simulink model "acc"  (R2021b)
settings: Solver=FixedStepAuto  StartTime=0.0  StopTime=206  FixedStep=0.0005  RelTol=1e-3
values from neighbouring files (symbols this model uses):
  Leftdis_PV_switch = 2    [acc_plot_backup.m]
  s_path = [0 1.10508939428 2.2141958029 3.32141571172 4.42705301151 5.53154548532 6.63517443471 7.73808041313 8.84055018688 9.94289959674 11.0453539299 12.1480581097 ... (1001 elements, 1001x1)]    [200_100radius.mat]    (also in LV_Clothoid_S_Turn_path.mat = [0 0.966832089581 1.93621320584 2.90214024471 3.86476766313 ; NEDC_path.mat = [0 0.414605943146 0.832514087334 1.25401518562 1.68216660344; Straight_East_into_curve.mat = [0 1.65770560069 3.32192925577 4.98420060507 6.64484613518 8; acc_plot_backup.m = Station_HV_m)
  X_path = [0 1.10508939428 2.2141958029 3.32141571172 4.42705301151 5.53154548532 6.63517443471 7.73808041313 8.84055018688 9.94289959674 11.0453539299 12.1480581097 ... (1001 elements, 1001x1)]    [200_100radius.mat]    (also in LV_Clothoid_S_Turn_path.mat = [-10 -9.03316791042 -8.06378679416 -7.09785975529 -6.1352323; NEDC_path.mat = [0 0.414605943146 0.832514087334 1.25401518562 1.68216660344; Straight_East_into_curve.mat = [0 1.65770560069 3.32192925577 4.98420060507 6.64484613518 8; acc_plot_backup.m = X_HV_m)
  Y_path = [0 -1.70364610795e-18 -7.41532896709e-18 1.46822109542e-17 4.74557362791e-17 6.12980216762e-17 9.25043977736e-17 1.24088240159e-16 1.5099156923e-16 1.7058517853e-16 1.90629227614e-16 2.09673434424e-16 ... (1001 elements, 1001x1)]    [200_100radius.mat]    (also in LV_Clothoid_S_Turn_path.mat = [0 -8.46153035536e-19 5.07382551045e-18 2.07356032218e-17 3.; NEDC_path.mat = [0 -3.50680326162e-18 -2.14111304971e-18 3.38197671014e-18 3; Straight_East_into_curve.mat = [0 1.29197709199e-18 2.81882429322e-18 3.49020462564e-17 6.7; acc_plot_backup.m = Y_HV_m)
undefined symbols (not defined in the file or in its folder): C_TICK_TIME_S, ENUM_ACCSTATE_DISABLED, ENUM_ACCSTATE_OFF, ENUM_ACCSTATE_STANDBY, FALSE, KVDI_ACCLongPressTime_ms, KVDI_ACCMaxActSpeed_kph, KVDI_ACCSetSpdIntial_kph, KVDI_ACCSpdLargeChange_kph, KVDI_LongPressConTime_ms, ONE_FLOAT, ONE_INT, R, Rw, T, TRUE, ZERO_FLOAT, ZERO_INT
libraries: simulink x16, dspstat3 x4, simulink_extras x2, Solver_SF x1
(part 4 of 4)

== matlab function acc/relative_dynamic_estimated/Measurement_update_X2 ==
  data: X_e input; u input; X_b output
function X_b=fcn(X_e,u)
T=0.01;
F=[1 T 0.5*T^2;0 1 T;0 0 1];
G=[-1/6*T^3;-1/2*T^2;-T];

X_b=F*X_e+G*u;
end

== matlab function acc/relative_dynamic_estimated/Time_update_X2 ==
  data: R input; Q input; K output; M2 output; M input
function [K,M2] = fcn(R,Q,M)
T=0.01;
% Rw=0.8;
% R=0.0001;
F=[1 T 0.5*T^2;0 1 T;0 0 1];
H=[1 0 0];
G=[-1/6*T^3;-1/2*T^2;-T];
G2=[1/6*T^3;1/2*T^2;T];

P=M-M*H'*inv(H*M*H'+R)*H*M;
% M2=F*P*F'+G2*Rw*G2';
M2=F*P*F'+Q;
K=P*H'*inv(R);
end

== matlab function acc/relative_dynamic_estimated/MATLAB Function3 ==
  data: X_b input; X_e output; K input; y input; d output; e output
function [X_e,d,e] = fcn(X_b,K,y)
H=[1 0 0];
d=y-H*X_b;
X_e=X_b+K*(y-H*X_b);
e=y-H*X_e;
end

== matlab function acc/relative_dynamic_estimated/MATLAB Function4 ==
  data: Q input; Q2 output; R input; M input; e input; d input; K input; R2 output; G output
function [Q2,R2,G] = fcn(Q,R,M,e,d,K)
a=0.9;
b=0.9;
H=[1 0 0];
R2=a*R+(1-a)*(e*e'+H*M*H');

Q2=b*Q+2*(1-b)*(K*d*d'*K');
G=0*Q+K*d*d*K';
end

== matlab function acc/relative_dynamic_estimated/Measurement_update_X3 ==
  data: X_e input; u input; X_b output
function X_b=fcn(X_e,u)
T=0.01;
F=[1 T 0.5*T^2;0 1 T;0 0 1];
G=[-1/6*T^3;-1/2*T^2;-T];

X_b=F*X_e+G*u;
end

== matlab function acc/relative_dynamic_estimated/Time_update_X3 ==
  data: R input; Q input; K output; M2 output; M input
function [K,M2] = fcn(R,Q,M)
T=0.01;
% Rw=0.8;
% R=0.0001;
F=[1 T 0.5*T^2;0 1 T;0 0 1];
H=[1 0 0];
G=[-1/6*T^3;-1/2*T^2;-T];
G2=[1/6*T^3;1/2*T^2;T];

P=M-M*H'*inv(H*M*H'+R)*H*M;
% M2=F*P*F'+G2*Rw*G2';
M2=F*P*F'+Q;
K=P*H'*inv(R);
end

== matlab function acc/Subsystem/longitudinal_driver_reference7 ==
  data: longitudinal_lane_refernce_trigger input; T input; Vxo input; Vxt input; ax_max input; jx_max input; Vx output; t output
function [Vx,t] = fcn(longitudinal_lane_refernce_trigger,T,Vxo,Vxt,ax_max,jx_max)
Vx=0;
Ax=0;
t=0;

if Vxt < Vxo
    ax_max=-ax_max;
    jx_max=-jx_max;
end

if longitudinal_lane_refernce_trigger==1

t1=ax_max/jx_max;
t2=(Vxt-Vxo)/ax_max;
t3=t1+t2;
t=T+0.1;


V1=Vxo+(0.5*jx_max*(t1^2));
V2=V1+(ax_max*(t2-t1));
   if t>=0 && t<=t1
       Ax=jx_max*t;
       Vx=double(Vxo+0.5*jx_max*(t^2));
   end
   if t>t1 && t<=t2
       Ax=ax_max;
       Vx=double(V1+(ax_max*(t-t1)));
   end
   if t>t2 && t<=t3
       Ax=ax_max-(jx_max*(t-t2));
       Vx=double(V2+ax_max*(t-t2)-0.5*jx_max*((t-t2)^2));
   end
   if t>t3
       Vx=double(Vxt);
       Ax=0;
   end
       

end
if longitudinal_lane_refernce_trigger==0
  Vx=double(Vxo);
 

   
end
end

== matlab function acc/Subsystem/longitudinal_driver_reference8 ==
  data: longitudinal_lane_refernce_trigger input; T input; Vxo input; Vxt input; ax_max input; jx_max input; Vx output; t output
function [Vx,t] = fcn(longitudinal_lane_refernce_trigger,T,Vxo,Vxt,ax_max,jx_max)
Vx=0;
Ax=0;
t=0;

if Vxt < Vxo
    ax_max=-ax_max;
    jx_max=-jx_max;
end

if longitudinal_lane_refernce_trigger==1

t1=ax_max/jx_max;
t2=(Vxt-Vxo)/ax_max;
t3=t1+t2;
t=T+0.1;


V1=Vxo+(0.5*jx_max*(t1^2));
V2=V1+(ax_max*(t2-t1));
   if t>=0 && t<=t1
       Ax=jx_max*t;
       Vx=double(Vxo+0.5*jx_max*(t^2));
   end
   if t>t1 && t<=t2
       Ax=ax_max;
       Vx=double(V1+(ax_max*(t-t1)));
   end
   if t>t2 && t<=t3
       Ax=ax_max-(jx_max*(t-t2));
       Vx=double(V2+ax_max*(t-t2)-0.5*jx_max*((t-t2)^2));
   end
   if t>t3
       Vx=double(Vxt);
       Ax=0;
   end
       

end
if longitudinal_lane_refernce_trigger==0
  Vx=double(Vxo);
 

   
end
end

== matlab function acc/Camera_NEW ==
  data: ux_mps input; phi_deg input; Xo input; Yo input; X_path parameter; s_path parameter; station input; x_ref output size=[22 1]; y_ref output size=[22 1]; Heading_ref output size=[22 1]; C output; Y_path parameter; Ts_MPC input
function [x_ref,y_ref,Heading_ref,C]  = Camera_emulator(ux_mps,phi_deg,Xo,Yo, X_path, s_path,station,Y_path, Ts_MPC)
% function [x_ref,y_ref,Y_path,Heading_ref,C]  = Camera_emulator(ux_mps,phi_deg,Xo,Yo, X_path, s_path,station,t_start,Ts_MPC,AES_pre_time,speed,Np,C0_Old, Y_path_Old)
% Path information is X_path, Y_path, s_path 
% Load path before running model===========================================
Np=22;
Tp=Ts_MPC*Np;

phi_rad=phi_deg*pi/180;

% global reference
% Yr=interp1(s_path,Y_path,station);
% path x,y body coordinate=================================================
x_path=cos(phi_rad)*(X_path-Xo)+sin(phi_rad)*(Y_path-Yo);
y_path=-sin(phi_rad)*(X_path-Xo)+cos(phi_rad)*(Y_path-Yo);
% current x,y body coordinate
% x_ref(1)=interp1(s_path,x_path,station);
% y_ref(1)=interp1(s_path,y_path,station);

s=ones(Np+2,1);
delta_s=Ts_MPC*ux_mps;
s=diag(0:Np+1)*s*delta_s+station;
%s=diag(-1:Np)*s*delta_s+station;

x_ref=zeros(Np,1);
y_ref=zeros(Np,1);
x_ref_12=interp1(s_path,x_path,s);
y_ref_12=interp1(s_path,y_path,s);
x_ref=x_ref_12(2:Np+1);
y_ref=y_ref_12(2:Np+1);
s_temp=s(Np)+Ts_MPC*ux_mps;

Heading_ref=zeros(Np,1);
for i=1:Np
    Heading_ref(i)=atan2(y_ref_12(i+2)-y_ref_12(i+1),x_ref_12(i+2)-x_ref_12(i+1));
end


%% CR=polyfit(x_R,y_R,3);
x=x_ref;
% Lane Change Module ======================================================

% if y_ref >= 1.5
%     y=y_ref-3.66;
% elseif y_ref <= -1.5
%     y=y_ref+3.66;
% else
%     y=y_ref+0;
% end
if y_ref >= 1.5
    y=y_ref-3.66;
elseif y_ref <= -1.5
    y=y_ref+3.66;
else
    y=y_ref+0;
end

%===================================================================
sum_x1=sum(x);
sum_x2=sum(x.^2);
sum_x3=sum(x.^3);
sum_x4=sum(x.^4);
sum_x5=sum(x.^5);
sum_x6=sum(x.^6);
sum_y=sum(y);
A=[length(x) sum_x1 sum_x2 sum_x3;
        sum_x1 sum_x2 sum_x3 sum_x4; 
        sum_x2 sum_x3 sum_x4 sum_x5; 
        sum_x3 sum_x4 sum_x5 sum_x6];
% A=[50 sum_x1 sum_x2 sum_x3;
%         sum_x1 sum_x2 sum_x3 sum_x4; 
%         sum_x2 sum_x3 sum_x4 sum_x5; 
%         sum_x3 sum_x4 sum_x5 sum_x6];
B=[sum_y;
      sum(x.*y);
      sum(x.*x.*y);
      sum(x.*x.*x.*y)];
% AES_pre_time=5;
% if Xo<=speed/3.6*(t_start-AES_pre_time)
%     C=[0; 0; 0; 0];
% else
    C=inv(A)*B;
% end
end

== matlab function acc/MPC_ACC ==
  data: trig input; vx_p input; u output; Vx input; ax input; Qs input; Rs input
function u = fcn(trig,vx_p,Vx,ax,Qs,Rs)
%% Initialzization
T = 0.1;
tau = 0.3;
Np = 10;
Nc = 3;

%% Mode Selector && MPC

A_spd = [1 T;0 1-T/tau];
B_spd = [0;T/tau];
C_spd = [1 0];

if trig == 1
    [m1,n1] = size(C_spd);
    h = zeros(Np,n1);
    F = zeros(Np,n1);
    h(1,:)=C_spd;
    F(1,:)=C_spd*A_spd;
    for j=2:Np
    h(j,:)=h(j-1,:)*A_spd; %Phi
    F(j,:)= F(j-1,:)*A_spd; 
    end
    v = h*B_spd;
    Phi_vx = zeros(Np,Nc);
    Phi_vx(:,1) = v;
    for k = 2:Nc
       Phi_vx(:,k) = [zeros(k-1,1);v(1:Np-k+1,1)]; %Toeplitz matrix
    end
    Q=Qs.*eye(Np); %Qw權重值=1;10
    R=Rs.*eye(Nc);%Rw權重值=0.07;1.5 ,0.07
    
    x_spd = [Vx;ax];
    Yref = vx_p';
    
    H = Phi_vx'*Q*Phi_vx+R;
    f = Phi_vx'*Q*(Yref-F*x_spd);
    U = inv(H)*f;
    u = U(1);

else
    u=0;
end
end

== matlab function acc/MATLAB Function5 ==
  data: u input; y output
function y = fcn(u)
persistent i;
if isempty(i)
    i = 1;
end

if i >=length(u)
    i=length(u);
end

y = u(i);
i = i+1;

== matlab function acc/MATLAB Function13 ==
  data: u input; y output
function y = fcn(u)
persistent i;
if isempty(i)
    i = 1;
end

if i >=length(u)
    i=length(u);
end

y = u(i);
i = i+1;

== matlab function acc/relative_dynamic_estimated/MATLAB Function6 ==
  data: X_b input; X_e output; K input; y input; d output; e output
function [X_e,d,e] = fcn(X_b,K,y)
H=[1 0 0];
d=y-H*X_b;
X_e=X_b+K*d;
e=y-H*X_e;
end

== matlab function acc/relative_dynamic_estimated/MATLAB Function7 ==
  data: Q input; Q2 output; R input; M input; e input; d input; K input; R2 output
function [Q2,R2] = fcn(Q,R,M,e,d,K)
a=0.5;
b=1;
H=[1 0 0];
R2=a*R+(1-a)*(e*e'+H*M*H');
if abs(d) < 0.02
    Q2=Q;
else
    Q2=b*Q+(1-b)*(K*d*d'*K');
end
end

== matlab function acc/relative_dynamic_estimated/Measurement_update_X5 ==
  data: X_e input; u input; X_b output
function X_b=fcn(X_e,u)
T=0.1;
F=[1 T 0.5*T^2;0 1 T;0 0 1];
G=[-1/6*T^3;-1/2*T^2;-T];

X_b=F*X_e+G*u;
end

== matlab function acc/relative_dynamic_estimated/Time_update_X5 ==
  data: R input; Q input; K output; M2 output; M input
function [K,M2] = fcn(R,Q,M)
T=0.1;
%% normal Kalman filter
% Rw=1; %變速度
% R=0.0001;
% Rw=0.5; %定速80
% R=0.001;
%% Adptive Kalman filter
%% 參數
F=[1 T 0.5*T^2;0 1 T;0 0 1];
H=[1 0 0];
G=[-(T^3)/6;-(T^2)/2;-T];
G2=[(T^3)/6;(T^2)/2;T];
%%
P=M-M*H'*inv(H*M*H'+R)*H*M;
% M2=F*P*F'+G2*Rw*G2';
M2=F*P*F'+Q;
K=P*H'*inv(R);
end

== matlab function acc/relative_dynamic_estimated/Q1 ==
  data: Rw output; d input; dx input; Rw1 input
function Rw  = fcn(d,dx,Rw1)
g=abs(d-dx);
if g > 0.04 && g< 0.5
    t=5;
elseif g <= 0.04 && g>0.02
    t=2;
else
    t=1;
end
if abs(d) > 0.002
    Rw=0.4*Rw1+0.6*abs(d^2)*10^t;
else
    Rw=Rw1*0.5;
end

end

== matlab function acc/relative_dynamic_estimated/R ==
  data: R output; e input; M input; R1 input
function R  = fcn(e,M,R1)
H=[1 0 0];
    R=(0.3*R1+0.7*(e*e+H*(M)*H'))/10;

end

== matlab function acc/relative_dynamic_estimated/Time_update_X6 ==
  data: Q input; R input; K output; P output; M2 output; M input
function [K,P,M2] = fcn(Q,R,M)
T=0.1;
% Rw=1; %變速度
% R=0.0001;
% Rw=1; %定速80
% R=0.001;
F=[1 T 0.5*T^2;0 1 T;0 0 1];
H=[1 0 0];
G=[-(T^3)/6;-(T^2)/2;-T];
G2=[(T^3)/6;(T^2)/2;T];

P=M-M*H'*inv(H*M*H'+R)*H*M;
M2=F*P*F'+G2*Q*G2';
% M2=F*P*F'+Q;
K=P*H'*inv(R);
end

== matlab function acc/relative_dynamic_estimated/Q ==
  data: Q output; d input; K input; Q1 input
function Q  = fcn(d,K,Q1)
if abs(d) > 0.002
    Q=0.3*Q1+0.7*(K*d*d*K');
else
    Q=Q1*0.9;
end

end

== matlab function acc/relative_dynamic_estimated/R2 ==
  data: R output; e input; M input; R1 input
function R  = fcn(e,M,R1)
H=[1 0 0];
% if e < 0.000001
%     R=R1;
% else
if abs(e)>0.1
    e=0.1;
end

% if abs(e) > 0.01
    R=0.3*R1+0.7*(e*e'+H*(M)*H');
%     R=0.3*R1+0.7*(e*e'+H*(M)*H')/;
% else
%     R=R1;
% end
% end
%     if R>0.01
%         R=0.01;
%     end
end

== matlab function acc/Subsystem/longitudinal_driver_reference9 ==
  data: longitudinal_lane_refernce_trigger input; T input; Vxo input; Vxt input; ax_max input; jx_max input; Vx output; t output
function [Vx,t] = fcn(longitudinal_lane_refernce_trigger,T,Vxo,Vxt,ax_max,jx_max)
Vx=0;
Ax=0;
t=0;

if Vxt < Vxo
    ax_max=-ax_max;
    jx_max=-jx_max;
end

if longitudinal_lane_refernce_trigger==1

t1=ax_max/jx_max;
t2=(Vxt-Vxo)/ax_max;
t3=t1+t2;
t=T+0.1;


V1=Vxo+(0.5*jx_max*(t1^2));
V2=V1+(ax_max*(t2-t1));
   if t>=0 && t<=t1
       Ax=jx_max*t;
       Vx=double(Vxo+0.5*jx_max*(t^2));
   end
   if t>t1 && t<=t2
       Ax=ax_max;
       Vx=double(V1+(ax_max*(t-t1)));
   end
   if t>t2 && t<=t3
       Ax=ax_max-(jx_max*(t-t2));
       Vx=double(V2+ax_max*(t-t2)-0.5*jx_max*((t-t2)^2));
   end
   if t>t3
       Vx=double(Vxt);
       Ax=0;
   end
       

end
if longitudinal_lane_refernce_trigger==0
  Vx=double(Vxo);
 

   
end
end

== matlab function acc/Estimation_TTCx_PV ==
  data: R input; TTC1 output; V input; A input; TTC2 output
function [TTC1,TTC2] = TTCx(R,V,A)
TTCp1=10;
TTCp2=10;
if R < 0
    R=-R;
    V=-V;
    A=-A;
end
% if R > 7
%     R=R-7;
% else
%     R=0;
% end
if R <= 0.1 % buff
    TTC1=0;
else
    if abs(A) > 1 && (V^2-2*A*R)>0
        TTCp1=(-V+sqrt(V^2-2*A*R))/A;
        TTCp2=(-V-sqrt(V^2-2*A*R))/A;
        if TTCp1>0 && TTCp2 >0
            TTC1 =min(TTCp1,TTCp2);
        elseif TTCp1 >= 0
            TTC1=TTCp1;
        else
            TTC1=TTCp2;
        end
    else
    TTC1=-R/V;
    end
end

if TTC1 > 10 
    TTC1=10;
end
if TTC1 < 0 
    TTC1=10;
end

if R < 0.1
    TTC2=0;
else
    TTC2=-R/V;
end
if  TTC2 > 10
    TTC2=10;
end
if  TTC2 < 0
    TTC2=10;
end
end

== matlab function acc/MPC_Bicycle_LDC1 ==
  data: trig input; Yref input; u output; Qs input; Rs input; Vy input; yaw_rate input; steer_angel input; Vx input; Ax input
function u  = fcn(trig,Yref,Qs,Rs,Vy,yaw_rate,steer_angel,Vx,Ax)
%% parameter
m=1501;
Caf=80.03*10^3;
Car=80.49*10^3;
Iz=1536.7; %2315
a=1.015;
b=1.895;
Np=10;
Nc=3;
tau=0.3;
T=0.1;
Y_ref=Yref;


if trig ==1


%% vehicle parameter

vx=zeros(Np,1);
vx(1)=Vx;
for z=2:Np
    vx(z)=vx(z-1)+Ax*T;
end

x_state = [0,Vy,0,yaw_rate,steer_angel]';



%% Vehicle Kinematics Model
% ----------------------------------------%
% x = [y, yaw angle, steering wheel angle]
% state row =5, state column =5,
%-----------------------------------------%
sr =5;
sc =5;
B = [0 0 0 0 (1/tau)*T]';
H = [1 0 0 0 0]; % [1, sr]

%% MPC parameter
% ------------------------------------------------------------------------------------------%
% Am is a vertor [A(k); A(k+1); A(k+2) ... A(k+np-1)]
% ------------------------------------------------------------------------------------------%
Am = zeros(sr, sc, Np);
for i = 1 : Np
    a13=vx(i)*T;
    a22=1-(Caf+Car)*T/(m*vx(i));
    a24=(b*Car-a*Caf)*T/(m*vx(i))-vx(i)*T;
    a25=Caf*T/m;
    a42=(b*Car-a*Caf)*T/(Iz*vx(i));
    a44=1-((a^2)*Caf+(b^2)*Car)*T/(Iz*vx(i));
    a45=a*Caf*T/Iz;
    a55=1-T/tau;
    Am(:,:,i)=[1 T a13 0 0;
        0 a22 0 a24 a25
        0 0 1 T 0
        0 a42 0 a44 a45
        0 0 0 0 a55];
end
% ------------------------------------------------------------------------------------------%
% Amm is a vector [A(k); A(k)A(k+1); A(k)A(k+1)A(k+2) ... A(k+np-1)]
% ------------------------------------------------------------------------------------------%
Amm = zeros(sr, sc, Np);
Amm(:, :, 1) = Am(:, :, 1);
for i = 2 : Np
    Amm(:, :, i) = Am(:, :, i) * Amm(:, :, i - 1);
end
% ----------------------------------------------------------------------------------------------%
% F is a metric [H A(k); H A(k)A(k+1); H A(k)A(k+1)A(k+2) ... H A(k+np-1)]
% size = [np, sc]
% ----------------------------------------------------------------------------------------------%
F = zeros(Np, sc);
for i = 1 : Np
    F(i, :) = H * Amm(:, : ,i);
end

% ----------------------------------------------------------------------------------------------%
% K is a metric [H A(k); H A(k)A(k+1); H A(k)A(k+1)A(k+2) ... H A(k+np-1)]
%size = [np nc]
%[H*B                                 0             0  ...       0  ]
%[H*A(k)*B                       H*B          0  ...        0 ] 
%[H*A(k)*A(k+1)*B       H*A(k)*B      0  ...    H*B ]
% the following quation is modified

%[H*B                                 0                   0          0          ...           0 ]
%[H*A(k+1)*B                          H*B                 0          0          ...           0 ] 
%[H*A(k+2)*A(k+1)*B                 H*A(k+2)*B           H*B         0          ...           0 ]
%[H*A(k+3)*A(k+2)*A(k+1)*B        H*A(k+3)*A(k+2)*B     H*A(k+3)*B   H*B        ...           0 ]
%[H*A(k+np-1)*A(k+np-2)*...*A(k+np-np+1)*B      H*A(k+np-1)*A(k+np-2)*...*A(k+np-np+2)*B     H*A(k+3)*B   H*B        ...           0 ]
% ----------------------------------------------------------------------------------------------%
K = zeros(Np, Nc);
K(1,1) = H*B;
for i = 2 : Np
    K(i,1) = F(i-1, :) * B;
end
for i = 2 : Nc
    K(i : Np, i) = K(i - 1 : Np - 1, i - 1);
end

%% final K
% K = eye(Np, Np);
% K = K * (H*B);
% Kmm = zeros(sr, sc, Np, Np);
% for i = 2 : Np
%     
%     Kmm(:, :, i, i-1) = Am(:, :, i);
%     K(i, i-1) = H * Kmm(:, :, i, i-1) * B;
% end
% 
% r = 1;
% for i = 3 : Np
%     Kmm(:, :, i, 1) = Am(:, :, i) * Kmm(:, :, i-1, 1);
%     K(i, 1) = H * Kmm(:, :, i, 1) * B;
%     m = i;
%     while (m >= 4 && m<=Np)
%         Kmm(:, :, m, r) = Am(:, :, m) * Kmm(:, :, m-1, r);
%         K(m, r) = H * Kmm(:, :, m, r) * B;
%         m = m+1;
%     end
%     r = r+1;
% end
% 
% if Nc ~= Np
%     K = K (1:Np, 1:Nc);
% end

% K = zeros(Np, Nc);
% K(1,1) = H*B;
% for i = 2 : Np
% end

% ----------------------------------------------------------------------------------------------%
%Q is the weighting of reference error
%R is the weighting of control gain
%our object is the minimize the cost function between these two option
% ----------------------------------------------------------------------------------------------%

Q = eye(Np);

Q = Q * Qs;
R = eye(Nc);
R = R * Rs;

% ----------------------------------------------------------------------------------------------%
%cost function
%J = (Rs - Y) * Q * (Rs - Y)' + U * R * U'
% after differential the cost function,and let dJ=0, we can get
%U = inv(K' * Q * K + R) * K' * Q * (rs - F * x_state)
%solve U, and the vector U is the optimal control gain series 

%when Rs == 2
%J = (Rs1 - Y1) * Q1 * (Rs1 - Y1)' + (Rs2 - Y2) * Q2 * (Rs2 - Y2)' + U * R * U'
%U = inv(K1' * Q * K1 + K2' * Q * K2 + R) * (K1' * Q1 * (Rs1 - F1 * x_state) + K2' * Q2 * (Rs2 - F2 * x_state))
% ----------------------------------------------------------------------------------------------%

U = inv(K' * Q * K + R) * K' * Q * (Y_ref - F * x_state);
u=U(1);

else
    u=0;
end
end

== stateflow chart acc/ACCSpdCalculation/Chart ==
  state INITIALIZATION
    en:
    NVDI_ACCSetSpd_kph = ZERO_INT;
    NVDI_ACCResSpd_kph=ZERO_INT;
    VVDI_ACCSpdDec_flg=FALSE;
    VVDI_ACCSpdInc_flg=FALSE;
  state STANDBY
    en:
    VVDI_ACCSpdDec_flg=FALSE;
    VVDI_ACCSpdInc_flg=FALSE;
    state Initial
      du:
      NVDI_ACCSetSpd_kph=NVDI_ACCSetSpdInitial_kph
    state Resume
      en:
      NVDI_ACCSetSpd_kph=NVDI_ACCResSpd_kph
    state Setting
      en:
      NVDI_ACCSetSpd_kph=NVDI_ACCSetSpdInitial_kph
    (default) -> Initial
    Initial -> Resume [order 2] : [VDINR_ACCSpdResInc_flg==TRUE...
        | &&NVDI_ACCResSpd_kph~=ZERO_INT]
    Resume -> Setting : [NVDI_SpdSet_flg==TRUE]
    Setting -> Resume : [VDINR_ACCSpdResInc_flg==TRUE...
        | &&NVDI_ACCResSpd_kph~=ZERO_INT]
    Initial -> Setting [order 1] : [NVDI_SpdSet_flg==TRUE]
  state SPEED_MODIF
    state Inc_Speed
      du:
      NVDI_ACCResSpd_kph=NVDI_ACCSetSpd_kph;
      VVDI_ACCSpdInc_flg=TRUE;
      state Small_Inc
        en:
        NVDI_ACCSetSpd_kph=NVDI_ACCSetSpd_kph+ONE_INT;
        NVDI_ACCIncTimer_ms=ZERO_INT;
        du:
        NVDI_ACCIncTimer_ms=NVDI_ACCIncTimer_ms+(C_TICK_TIME_S*1000);
      state Large_Inc_Frist
        en:
        NVDI_ACCSetSpd_kph=NVDI_LongPressSpdIntial_kph+KVDI_ACCSpdLargeChange_kph
      state MAINTAIN
        en:
        NVDI_ACCIncTimer_ms=ZERO_INT;
        du:
        NVDI_ACCIncTimer_ms=NVDI_ACCIncTimer_ms+(C_TICK_TIME_S*1000);
      state Large_Inc
        en:
        NVDI_ACCSetSpd_kph=NVDI_ACCSetSpd_kph+KVDI_ACCSpdLargeChange_kph
      (default) -> Small_Inc
      Small_Inc -> Large_Inc_Frist : [NVDI_ACCIncTimer_ms>KVDI_ACCLongPressTime_ms]
      Large_Inc_Frist -> SPEED_MODIF.Inc_Speed.MAINTAIN
      SPEED_MODIF.Inc_Speed.MAINTAIN -> Large_Inc : [NVDI_ACCIncTimer_ms>KVDI_LongPressConTime_ms]
      Large_Inc -> SPEED_MODIF.Inc_Speed.MAINTAIN
    state Dec_Speed
      du:
      NVDI_ACCResSpd_kph=NVDI_ACCSetSpd_kph;
      VVDI_ACCSpdDec_flg=TRUE;
      state Small_Dec
        en:
        NVDI_ACCSetSpd_kph=NVDI_ACCSetSpd_kph-ONE_INT;
        NVDI_ACCDecTimer_ms=ZERO_INT;
        du:
        NVDI_ACCDecTimer_ms=NVDI_ACCDecTimer_ms+(C_TICK_TIME_S*1000);
      state Large_Dec_Frist
        en:
        NVDI_ACCSetSpd_kph=NVDI_LongPressSpdIntial_kph
      state MAINTAIN
        en:
        NVDI_ACCDecTimer_ms=ZERO_INT;
        du:
        NVDI_ACCDecTimer_ms=NVDI_ACCDecTimer_ms+(C_TICK_TIME_S*1000);
      state Large_Dec
        en:
        NVDI_ACCSetSpd_kph=NVDI_ACCSetSpd_kph-KVDI_ACCSpdLargeChange_kph
      (default) -> Small_Dec
      Small_Dec -> Large_Dec_Frist : [NVDI_ACCDecTimer_ms>KVDI_ACCLongPressTime_ms]
      Large_Dec_Frist -> SPEED_MODIF.Dec_Speed.MAINTAIN
      Large_Dec -> SPEED_MODIF.Dec_Speed.MAINTAIN
      SPEED_MODIF.Dec_Speed.MAINTAIN -> Large_Dec : [NVDI_ACCDecTimer_ms>KVDI_LongPressConTime_ms]
    state HOLD
      en:
      NVDI_ACCSetSpd_kph=NVDI_ACCSetSpd_kph
      NVDI_ACCResSpd_kph=NVDI_ACCSetSpd_kph;
      VVDI_ACCSpdDec_flg=FALSE;
      VVDI_ACCSpdInc_flg=FALSE;
    (default) -> HOLD
    HOLD -> Dec_Speed [order 1] : [VDINR_ACCSpdSetDec_flg==TRUE]
    HOLD -> Inc_Speed [order 2] : [VDINR_ACCSpdResInc_flg==TRUE]
    Dec_Speed -> HOLD : [VDINR_ACCSpdSetDec_flg==FALSE]
    Inc_Speed -> HOLD : [VDINR_ACCSpdResInc_flg==FALSE]
  (default) -> INITIALIZATION
  INITIALIZATION -> STANDBY : [NVDI_ACCSystemStatePrev_enum == ENUM_ACCSTATE_STANDBY]
  STANDBY -> SPEED_MODIF [order 2] : [NVDI_ACCActingPrev_flg==TRUE]
  STANDBY -> INITIALIZATION [order 1] : [NVDI_ACCSystemStatePrev_enum == ENUM_ACCSTATE_OFF...
      | || NVDI_ACCSystemStatePrev_enum == ENUM_ACCSTATE_DISABLED]
  SPEED_MODIF -> STANDBY [order 2] : [NVDI_ACCActingPrev_flg==FALSE]
  SPEED_MODIF -> INITIALIZATION [order 1] : [NVDI_ACCSystemStatePrev_enum == ENUM_ACCSTATE_OFF...
      | || NVDI_ACCSystemStatePrev_enum == ENUM_ACCSTATE_DISABLED]
  data: NVDI_SpdSet_flg input; VDINR_ACCSpdSetDec_flg input; VDINR_ACCSpdResInc_flg input; NVDI_ACCSetSpdInitial_kph input; NVDI_ACCActingPrev_flg input; NVDI_ACCSystemStatePrev_enum input; NVDI_ACCSetSpd_kph output; KVDI_ACCLongPressTime_ms input; NVDI_LongPressSpdIntial_kph input; TRUE parameter boolean; ZERO_INT parameter; ONE_INT parameter; FALSE parameter boolean; ENUM_ACCSTATE_STANDBY parameter; ENUM_ACCSTATE_OFF parameter; ENUM_ACCSTATE_DISABLED parameter; C_TICK_TIME_S parameter; NVDI_ACCIncTimer_ms local; NVDI_ACCDecTimer_ms local; KVDI_ACCSpdLargeChange_kph parameter; NVDI_ACCResSpd_kph local; VVDI_ACCSpdInc_flg output; VVDI_ACCSpdDec_flg output; KVDI_LongPressConTime_ms input

== matlab function acc/MATLAB Function10 ==
  data: RR input; RX output; RD input; RY output
function [RX,RY] = fcn(RR,RD)
RX=RR*cosd(RD);
RY=RR*sind(RD);
end

== matlab function acc/Smooth Switch/MATLAB Function ==
  data: tau input; u input; y output; old_u input
function y = fcn(tau,u,old_u)

T=0.1; % sample time

y=u*(T/(tau+T))+old_u*(tau/(tau+T));


end

== matlab function acc/MPC ==
  data: vx_p input; vx_acc_set input; mode input; vxh input; axh input; HH output; X_thk input; ax_c_old input; ff output; M_act output; gamma_act output; fesible_flag output
function [HH,ff,M_act,gamma_act,fesible_flag] = fcn(vx_p,vx_acc_set,mode,vxh,axh,X_thk,ax_c_old)
%% Initialzization
a=1.1135; l=2.62; b=l-a; 
g=9.81; 
m=1660+22*4; 

vx_p_th = zeros(1,10);
% actuator dynamics
tau_a = 0.3; 
% desired time headway
TH = 1.5;
% Prediction horizon
Np = 10 ;
% Control horizon
Nc = 5;
T = 0.1;
% soft constraint related
rho = 3*eye(1); % weight for slakes
epsilon1 = 0.3;  % slake for time heaway
epsilon2 = 1;  % slake for vehicle velocity
% states
X_xk = [vxh;axh;ax_c_old];
Ax = X_thk(3);
% axMFV = axh + Ax;

%% Three modes
Rx = X_thk(1);
if (Rx <= 2) && (mode == 2)
    mode = 3;
end

if mode == 1 % Speed control mode
    
    Xk = X_xk; % Xk = [vx,ax,delta_ax_c_old]
    phi_x = [ 1 T;
              0 1-(T/tau_a)];
    gamma_x = [0 T/tau_a]';
    H=[1 0 0];
    H1 = [0 1 0];
    phi=[phi_x gamma_x;0 0 1];
    gamma=[gamma_x; 1];

    Number_state = 3;
    
    Rs = vx_p(1:10,1); % Colume vector

elseif mode == 2 % TH control mode
    
    Xk = X_thk; % Xk = [Rx,Vx,Ax,ax_a, delta_ax]
    phi_x = [ 1 T 0.5*T^2+T^3/6 0 -T^3/6;
           0 1 T+0.5*T^2 0 0.5*T^2;
          0 0 1 0 T/tau_a;
          0 0 0 1 T;
          0 0 0 0 1-T/tau_a];
    gamma_x = [-(1/6)*T^3 -0.5*T^2 -T/tau_a 0 T/tau_a]';
    H=[1 0 0 0 0 0];
    H1 = [0 0 0 1 0 0];
    phi=[phi_x gamma_x;0 0 0 0 0 1];
    gamma=[gamma_x; 1];

    Number_state = 6;
    vx_p_th_buf = vxh;
    for i1 = 1:Np
        t = i1*T;
        vx_p_th(i1) = vx_p_th_buf;
        vx_p_th_buf = vx_p_th_buf + axh*t;
    end
    Rth = TH*vx_p_th; % ref relative distance
    Rs = Rth'; % colume vector
else    

    Xk = X_xk; % Xk = [vx,ax,delta_ax_c_old]
    phi_x = [ 1 T;
              0 1-(T/tau_a)];
    gamma_x = [0 T/tau_a]';
    H=[1 0 0];
    H1 = [0 1 0];
    phi=[phi_x gamma_x;0 0 1];
    gamma=[gamma_x; 1];

    Number_state = 3;
    
    Rs = (vx_acc_set)*ones(Np,1); % colume vector
 
end



F = zeros(Np,Number_state);
K = zeros(Np,Nc);
F1 = zeros(Np,Number_state);
K1 = zeros(Np,Nc);
buf_p = zeros(1,Nc);
%% Prediction model

for i = 1:Np
    F(i,1:Number_state)=H*phi^i;
    K(i,1)=H*(phi^(i-1))*gamma;
end

for j = 2:Nc
    K(j,j)=K(1);
end

for i = 3:Np
    if i < Nc
        buf = fliplr(K(2:i-1,1)');
        K(i,2:(i-1))=buf;
    else
        for j = 1:Nc
            buf_p(1,j) = H*(phi^(j+i-Nc-1))*gamma;
        end
%         buf = fliplr(K(i+1:i+Nc-1,1)');
        K(i,1:Nc)=fliplr(buf_p);       
    end
end

% vehicle velocity
for i = 1:Np
    F1(i,1:Number_state)=H1*phi^i;
    K1(i,1)=H1*(phi^(i-1))*gamma;
end

for j = 2:Nc
    K1(j,j)=K(1);
end

for i = 3:Np
    if i < Nc
        buf = fliplr(K(2:i-1,1)');
        K1(i,2:(i-1))=buf;
    else
        for j = 1:Nc
            buf_p(1,j) = H1*(phi^(j+i-Nc-1))*gamma;
        end
%         buf = fliplr(K(i+1:i+Nc-1,1)');
        K1(i,1:Nc)=fliplr(buf_p);       
    end
end

%% MPC constraints
C1 = ones(Nc,1);
C2 = tril(ones(Nc));
% amplitude constraint on control signal
Umin = -2*ones(Nc,1);
Umax = 2*ones(Nc,1);
% increment constraint on control signal
deltaU_min = -1.5*ones(Nc,1);
deltaU_max = 1.5*ones(Nc,1);
% % amplitude constraint on ralative distance defined by time headway
% Y_min = -()*ones(Np,1);
Rx_min = (vxh*(1.))*ones(Np,1);
Rx_max =(vxh*(TH+0.5))*ones(Np,1);
% % amplitude constraint on vehicle velocity
vx_min = 30/3.6*ones(Np,1);
vx_max =100/3.6*ones(Np,1);

M1 = [-C2;C2];
N1 = [-Umin+C1*ax_c_old; Umax-C1*ax_c_old];
M2=[-eye(Nc,Nc); eye(Nc,Nc)];
N2 = [-deltaU_min; deltaU_max];
M3 = [-K;K];
N3 = [-Rx_min+F*Xk; Rx_max-F*Xk];
M4 = [-K;K];
N4 = [-vx_min+F1*Xk; vx_max-F1*Xk];

% M_slake = [zeros(Nc*4,1) ; epsilon*ones(Np*2,1);-epsilon*ones(Np*2,1)];
M_slake1 = [zeros(Nc*4,1); 
    epsilon1*ones(Np,1);
    -epsilon1*ones(Np,1)
    zeros(Np,1);
    zeros(Np,1)];
M_slake2 = [zeros(Nc*4,1); 
%     zeros(Np,1);
%     zeros(Np,1);
    epsilon2*ones(Np,1);
    -epsilon2*ones(Np,1)];
% M_slake = [zeros(Nc*4,1)];

M = [M1; M2;M4];
gamma_act = [N1; N2;N4];
M_act = [M,M_slake2];
% M_act = [M,M_slake1,M_slake2];
% M_act = M;

%% Transform to QP form 
Q=1.*eye(Np);
R_bar=0.2*eye(Nc);

HH_buf = [K'*Q*K + R_bar,zeros(Nc,1);
    zeros(1,Nc), rho];
ff = [-2*K'*Q*(Rs-F*Xk);0];
HH = (HH_buf + HH_buf')/2;
% determine if the problem is fesible
eig_vals  = eig(HH); 
fesible_flag = [sum([sign(eig_vals)==1])==length(HH)];

== matlab function acc/QP_logitudinal1 ==
  data: u output; H input; f input; A_cons input; b input; u_old input
function u =QPhild(H,f,A_cons, b,u_old)
% E=H;
% F=f;
% M=A_cons;
% gamma=b;
% eta =x
% u_star = zeros(1);
% aa = ones(1);
[n1,m1]=size(A_cons);
% eta=H\f;
% kk=0;
% for i=1:n1
%     if (A_cons(i,:)*eta>b(i)) kk=kk+1;
%     else
%     kk=kk+0;
%     end
% end

% if (kk==0) return; end

P=A_cons*(H\A_cons');
d=(A_cons*(H\f)+b);
[n,m]=size(d);
x_ini=zeros(n,m);
lambda=x_ini;
al=10;

for km=1:25   %% P68
%     find the elements in the solution vector one by one
%     km could be larger if the Lagranger multiplier has a slow
%     convergence rate.
    lambda_p=lambda;
    for i=1:n
        w= P(i,:)*lambda-P(i,i)*lambda(i,1);
        w=w+d(i,1);
        la=-w/P(i,i);
        lambda(i,1)=max(0,la);
    end
    al=(lambda-lambda_p)'*(lambda-lambda_p);

    if (al<10e-8); break; end
end
eta=-H\f -H\A_cons'*lambda;

% eta=inv(H)*f;
% if isempty(eta)     %eta
%     [n1,m1]=size(A_cons_soft1);
%     eta1=-H\f;
%     kk=0;
%     for i=1:n1
%         if (A_cons_soft1(i,:)*eta1>b_soft1(i)) kk=kk+1;
%         else
%         kk=kk+0;
%         end
%     end
% 
%     if (kk==0) return; end
% 
%     P=A_cons_soft1*(H\A_cons_soft1');
%     d=(A_cons_soft1*(H\f)+b_soft1);
%     [n,m]=size(d);
%     x_ini=zeros(n,m);
%     lambda=x_ini;
%     al=10;
% 
%     for km=1:38
%         %find the elements in the solution vector one by one
%         % km could be larger if the Lagranger multiplier has a slow
%         % convergence rate.
%         lambda_p=lambda;
%         for i=1:n
%             w= P(i,:)*lambda-P(i,i)*lambda(i,1);
%             w=w+d(i,1);
%             la=-w/P(i,i);
%             lambda(i,1)=max(0,la);
%         end
%         al=(lambda-lambda_p)'*(lambda-lambda_p);
% 
%         if (al<10e-8); break; end
%     end
%     eta1=-H\f -H\A_cons_soft1'*lambda;
%     if isempty(eta1) %eta1
%         [n1,m1]=size(A_cons_soft2);
%         eta2=-H\f;
%         kk=0;
%         for i=1:n1
%             if (A_cons_soft2(i,:)*eta2>b_soft2(i)) kk=kk+1;
%             else
%             kk=kk+0;
%             end
%         end
% 
%         if (kk==0) return; end
% 
%         P=A_cons_soft2*(H\A_cons_soft2');
%         d=(A_cons_soft2*(H\f)+b_soft2);
%         [n,m]=size(d);
%         x_ini=zeros(n,m);
%         lambda=x_ini;
%         al=10;
% 
%         for km=1:38
%             %find the elements in the solution vector one by one
%             % km could be larger if the Lagranger multiplier has a slow
%             % convergence rate.
%             lambda_p=lambda;
%             for i=1:n
%                 w= P(i,:)*lambda-P(i,i)*lambda(i,1);
%                 w=w+d(i,1);
%                 la=-w/P(i,i);
%                 lambda(i,1)=max(0,la);
%             end
%             al=(lambda-lambda_p)'*(lambda-lambda_p);
% 
%             if (al<10e-8); break; end
%         end
%         eta2=-H\f -H\A_cons_soft2'*lambda;
%         u_star = eta2(1);
%     else
%         u_star = eta1(1);
%     end
% else
    aa = lambda(1);
    xk = eta(1);
    u=eta(1)+u_old;
end

== matlab function acc/cmd_limiter2/Smooth Switch/MATLAB Function ==
  data: tau input; u input; y output; old_u input
function y = fcn(tau,u,old_u)

T=0.1; % sample time

y=u*(T/(tau+T))+old_u*(tau/(tau+T));


end

== matlab function acc/cmd_limiter3/Smooth Switch/MATLAB Function ==
  data: tau input; u input; y output; old_u input
function y = fcn(tau,u,old_u)

T=0.1; % sample time

y=u*(T/(tau+T))+old_u*(tau/(tau+T));


end

== matlab function acc/Kalman_Filter_LatSpd1 ==
  data: X_e output; X_e input; u input; Yaw_rate input; R input; Q input; y input; X_k output; F output; G output; G2 output; K output; M input; M2 output
function [X_e,X_k,F,G,G2,K,M2] = fcn(X_e,u,Yaw_rate,R,Q,y,M)
t= 0.1;

r_th= 0.015;

F = [1 Yaw_rate*t;
     -Yaw_rate*t 1];

G = [t 0;0 t];

G2 = [-X_e(2)*t -t 0;
       X_e(1)*t 0 -t];
X_k = F*X_e+G*u;
% X_k = F*X_e;
%%
Rn = R;
Qn = Q*[0.01 0 0;
       0 100 0;
       0 0 0.01];
H = [1 0];
P = M-M*H'*inv(H*M*H'+Rn)*H*M;
M2 = F*P*F'+G2*Qn*G2';
if abs(Yaw_rate)>=r_th
    K=P*H'*inv(Rn);
else
    K = zeros(2,1);
end
X_e=X_k+K*(y-H*X_k);
end

== matlab function acc/MATLAB Function4 ==
  data: RR input; RX output; RD input; RY output
function [RX,RY] = fcn(RR,RD)
RX=RR*cosd(RD);
RY=RR*sind(RD);
end

== matlab function acc/MATLAB Function6 ==
  data: Xf input; RR output; Yf input; Xh input; Yh input; RD output
function [RR,RD] = fcn(Xf,Yf,Xh,Yh)
RX=Xf-Xh;
RY=Yf-Yh;
if RX >= 0
    RR=sqrt(RX^2+RY^2);
    RD=atand(RY/RX);
else
    RR=sqrt(RX^2+RY^2);
    RD=atand(RY/RX)+180;
end
% if RD < -0.1
%     RD=RD+360;
% end
end

== matlab function acc/LateralMotionKF1 ==
  data: T input; rk input; vxk input; delta input; Caf input; Car input; lf input; lr input; vyk1 output; mv input; vyk input; ayk output
function [vyk1,ayk] = fcn(T,rk,vxk,delta,Caf,Car,lf,lr,mv,vyk)
%%
if vxk >= 15/3.6
    ayk = -(Caf*( atan( (vyk+lf*rk)/vxk -delta) ) + Car*atan((vyk-lr*rk)/vxk))/mv;
else
    ayk = 0;
end

vyk1 = vyk-T*rk*vxk + T*ayk;
% vyk1 =T*ayk;

== matlab function acc/Estimation_TTCx_PV1 ==
  data: R input; TTC1 output; V input; A input; TTC2 output
function [TTC1,TTC2] = TTCx(R,V,A)
TTCp1=10;
TTCp2=10;
if R < 0
    R=-R;
    V=-V;
    A=-A;
end
% if R > 7
%     R=R-7;
% else
%     R=0;
% end
if R <= 0.1 % buff
    TTC1=0;
else
    if abs(A) > 1 && (V^2-2*A*R)>0
        TTCp1=(-V+sqrt(V^2-2*A*R))/A;
        TTCp2=(-V-sqrt(V^2-2*A*R))/A;
        if TTCp1>0 && TTCp2 >0
            TTC1 =min(TTCp1,TTCp2);
        elseif TTCp1 >= 0
            TTC1=TTCp1;
        else
            TTC1=TTCp2;
        end
    else
    TTC1=-R/V;
    end
end

if TTC1 > 10 
    TTC1=10;
end
if TTC1 < 0 
    TTC1=10;
end

if R < 0.1
    TTC2=0;
else
    TTC2=-R/V;
end
if  TTC2 > 10
    TTC2=10;
end
if  TTC2 < 0
    TTC2=10;
end
end

== matlab function acc/MATLAB Function7 ==
  data: OnlyPV_signal input; RR_PV input; RR output; RV output; RA output; RR_APV input; RVx_PV input; RVx_APV input; RAx_PV input; RAx_APV input; RY_PV input; RY_APV input; RD_PV input; RD_APV input; trig output
function [RR,RV,RA,trig] = fcn(OnlyPV_signal,RR_PV,RR_APV,RVx_PV,RVx_APV,RAx_PV,RAx_APV,RY_PV,RY_APV,RD_PV,RD_APV)
if OnlyPV_signal==0
    if RR_APV < RR_PV && RY_APV-RY_PV <= 0.3 && RD_APV-RD_PV <= 5
        
        RR=RR_APV;
        RV=RVx_APV;
        RA=RAx_APV;
        trig=1;
    else
    
        RR=RR_PV;
        RV=RVx_PV;
        RA=RAx_PV;
        trig=0;
    end
else
    RR=RR_PV;
    RV=RVx_PV;
    RA=RAx_PV;
    trig=0;
end

end

== matlab function acc/Estimation_TTCx_PV2 ==
  data: R input; TTC1 output; V input; A input; TTC2 output
function [TTC1,TTC2] = TTCx(R,V,A)
up_bound=10;
TTCp1=up_bound;
TTCp2=up_bound;
if R < 0
    R=-R;
    V=-V;
    A=-A;
end
% if R > 7
%     R=R-7;
% else
%     R=0;
% end
if R <= 0.1 % buff
    TTC1=0;
else
    if abs(A) > 1 && (V^2-2*A*R)>0
        TTCp1=(-V+sqrt(V^2-2*A*R))/A;
        TTCp2=(-V-sqrt(V^2-2*A*R))/A;
        if TTCp1>0 && TTCp2 >0
            TTC1 =min(TTCp1,TTCp2);
        elseif TTCp1 >= 0
            TTC1=TTCp1;
        else
            TTC1=TTCp2;
        end
    else
    TTC1=-R/V;
    end
end

if TTC1 > up_bound
    TTC1=up_bound;
end
if TTC1 < 0 
    TTC1=up_bound;
end

if R < 0.1
    TTC2=0;
else
    TTC2=-R/V;
end
if  TTC2 > up_bound
    TTC2=up_bound;
end
if  TTC2 < 0
    TTC2=up_bound;
end
end

== matlab function acc/Cut-in strategy/MATLAB Function11 ==
  data: tau input; u input; y output; old_u input
function y = fcn(tau,u,old_u)

T=0.1; % sample time

y=u*(T/(tau+T))+old_u*(tau/(tau+T));


end
